simulink model "LAB_Stima_e_Controllo_Lez_3_Sistema_Idraulico_Simulink"  (R2018a)
settings: Solver=ode45  StartTime=0.0  StopTime=1000.0  RelTol=1e-3
values from neighbouring files (symbols this model uses):
  A = [0 1 0;0 -f/J km/J;0 -kv/La -Ra/La]    [LAB_Stima_e_Controllo_Lez_1_Motore_Corrente_Continua.m]    (also in LAB_Stima_e_Controllo_Lez_2_Sistema_Idraulico.m = [-a a 0;a -2*a a;0 a -(a+b)]; LAB_Stima_e_Controllo_Lez_4_Pendolo_Inverso.m = [0 1 0 0;0 0 -(m*g)/M 0;0 0 0 1;0 0 ((M+m)*g)/(M*L) 0]; LAB_Stima_e_Controllo_Lez_6_Filtro_di_Kalman_TC.m; LAB_Stima_e_Controllo_Lez_6_Filtro_di_Kalman_TD.m = [1.1269 -0.4940 0.1129;1 0 0;0 1 0])
  A0 = A-L*C    [LAB_Stima_e_Controllo_Lez_2_Sistema_Idraulico.m]
  B = [0;0;Ga/La]    [LAB_Stima_e_Controllo_Lez_1_Motore_Corrente_Continua.m]    (also in LAB_Stima_e_Controllo_Lez_2_Sistema_Idraulico.m = [1/S 0;0 0;0 1/S]; LAB_Stima_e_Controllo_Lez_4_Pendolo_Inverso.m = [0;1/M;0;-1/(M*L)]; LAB_Stima_e_Controllo_Lez_6_Filtro_di_Kalman_TC.m; LAB_Stima_e_Controllo_Lez_6_Filtro_di_Kalman_TD.m = [-0.3832;0.5919;0.5191])
  C = [1 0 0]    [LAB_Stima_e_Controllo_Lez_1_Motore_Corrente_Continua.m]    (also in LAB_Stima_e_Controllo_Lez_2_Sistema_Idraulico.m = [0 0 1]; LAB_Stima_e_Controllo_Lez_4_Pendolo_Inverso.m = [1 0 0 0;0 0 1 0]; LAB_Stima_e_Controllo_Lez_6_Filtro_di_Kalman_TC.m; LAB_Stima_e_Controllo_Lez_6_Filtro_di_Kalman_TD.m)
  D = 0    [LAB_Stima_e_Controllo_Lez_1_Motore_Corrente_Continua.m]    (also in LAB_Stima_e_Controllo_Lez_2_Sistema_Idraulico.m = [0 0]; LAB_Stima_e_Controllo_Lez_4_Pendolo_Inverso.m; LAB_Stima_e_Controllo_Lez_6_Filtro_di_Kalman_TC.m; LAB_Stima_e_Controllo_Lez_6_Filtro_di_Kalman_TD.m)
  h1 = 11    [LAB_Stima_e_Controllo_Lez_2_Sistema_Idraulico.m]
  h2 = 9    [LAB_Stima_e_Controllo_Lez_2_Sistema_Idraulico.m]
  h3 = 6    [LAB_Stima_e_Controllo_Lez_2_Sistema_Idraulico.m]
  K1 = place(A,B,p1)    [LAB_Stima_e_Controllo_Lez_1_Motore_Corrente_Continua.m]    (also in LAB_Stima_e_Controllo_Lez_2_Sistema_Idraulico.m; LAB_Stima_e_Controllo_Lez_4_Pendolo_Inverso.m)
  L = KD'    [LAB_Stima_e_Controllo_Lez_2_Sistema_Idraulico.m]    (also in LAB_Stima_e_Controllo_Lez_4_Pendolo_Inverso.m = 0.5)
  q10 = 1    [LAB_Stima_e_Controllo_Lez_2_Sistema_Idraulico.m]
  q30 = 0.5    [LAB_Stima_e_Controllo_Lez_2_Sistema_Idraulico.m]
settings Model: Creator=anton  LastModifiedBy=anton

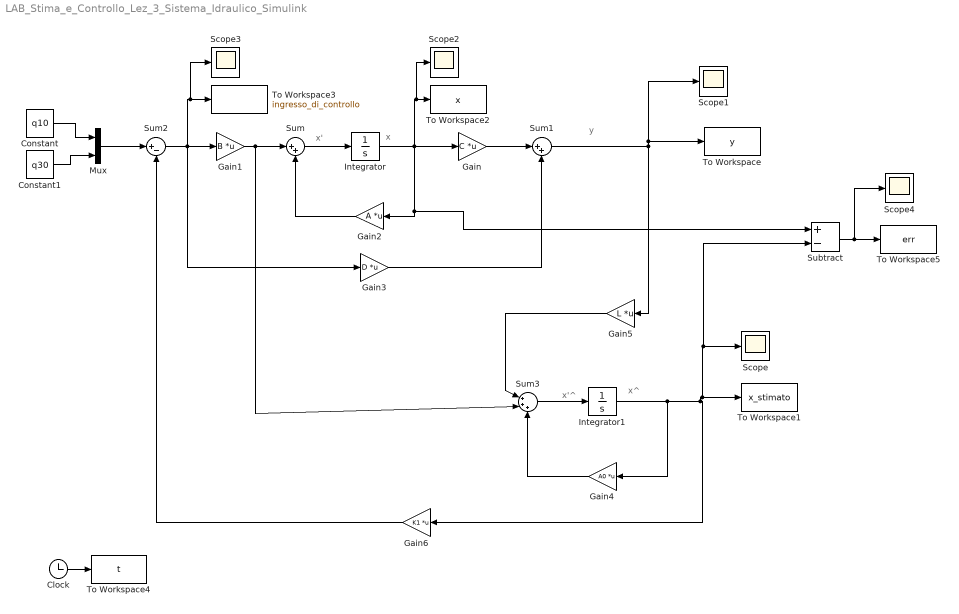
== system LAB_Stima_e_Controllo_Lez_3_Sistema_Idraulico_Simulink ==
  note: x^
  note: x'^
  note: y
  note: x
  note: x'
  Clock : Clock
  Constant : Constant  Value=q10
  Constant1 : Constant  Value=q30
  Gain : Gain  Gain=C  Multiplication=Matrix(K*u)
  Gain1 : Gain  Gain=B  Multiplication=Matrix(K*u)
  Gain2 : Gain  Gain=A  Multiplication=Matrix(K*u)
  Gain3 : Gain  Gain=D  Multiplication=Matrix(K*u)
  Gain4 : Gain  Gain=A0  Multiplication=Matrix(K*u)
  Gain5 : Gain  Gain=L  Multiplication=Matrix(K*u)
  Gain6 : Gain  Gain=K1  Multiplication=Matrix(K*u)
  Integrator : Integrator  InitialCondition=[h1;h2;h3]
  Integrator1 : Integrator  InitialCondition=[h1+1;h2-1;h3+2]
  Mux : Mux  Inputs=2
  Scope{,1..4} (5 alike) : Scope
  Subtract : Sum  Inputs=+-
  Sum : Sum  Inputs=|++
  Sum1 : Sum  Inputs=|++
  Sum2 : Sum  Inputs=|+-
  Sum3 : Sum  Inputs=|+++
  To Workspace : ToWorkspace  VariableName=y  SampleTime=-1
  To Workspace1 : ToWorkspace  VariableName=x_stimato  SampleTime=-1
  To Workspace2 : ToWorkspace  VariableName=x  SampleTime=-1
  To Workspace3 : ToWorkspace  VariableName=ingresso_di_controllo  SampleTime=-1
  To Workspace4 : ToWorkspace  VariableName=t  SampleTime=-1
  To Workspace5 : ToWorkspace  VariableName=err  SampleTime=-1
  wires:
  Gain1/1 -> Sum3/2, Sum/1
  Sum/1 -> Integrator/1
  Integrator/1 -> Scope2/1, To Workspace2/1, Subtract/1, Gain2/1, Gain/1
  Gain2/1 -> Sum/2
  Sum2/1 -> Scope3/1, To Workspace3/1, Gain3/1, Gain1/1
  Gain/1 -> Sum1/1
  Gain3/1 -> Sum1/2
  Sum1/1 -> Scope1/1, To Workspace/1, Gain5/1
  Gain5/1 -> Sum3/1
  Sum3/1 -> Integrator1/1
  Gain4/1 -> Sum3/3
  Integrator1/1 -> Gain4/1, Subtract/2, Scope/1, To Workspace1/1, Gain6/1
  Gain6/1 -> Sum2/2
  Mux/1 -> Sum2/1
  Constant1/1 -> Mux/2
  Constant/1 -> Mux/1
  Clock/1 -> To Workspace4/1
  Subtract/1 -> Scope4/1, To Workspace5/1
